simulink model "constantTorqueDemo"  (Simulink 8.3)
settings: Solver=ode45  StartTime=0.0  StopTime=inf  RelTol=1e-3
undefined symbols (not defined in the file or in its folder): PendulumPlant, PendulumVisualizer
libraries: drake x3, simulink x3
settings Model: Creator=russt  LastModifiedBy=russt
settings OptimizationCC: ExpressionDepthLimit=2147483647
settings DebuggingCC: FcnCallInpInsideContextMsg=UseLocalSettings

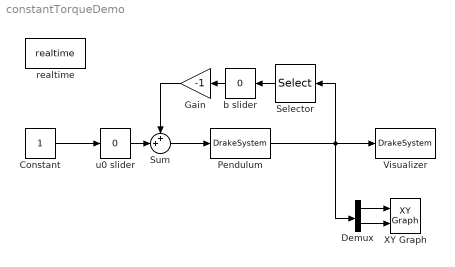
== system constantTorqueDemo ==
  Constant : Constant
  Demux : Demux  Outputs=2
  Gain : Gain  Gain=-1
  Pendulum : drake/DrakeSystem  sysobj=PendulumPlant(0)
  Selector : Selector  InputPortWidth=2  Indices=2
  Sum : Sum  Inputs=++|
  Visualizer : drake/DrakeSystem  sysobj=PendulumVisualizer()
  XY Graph : simulink/Sinks/XY Graph  xmin=-pi  xmax=pi  ymin=-4  ymax=4  st=-1
  "b slider " : simulink/Math Operations/Slider Gain  low=-5  gain=0  high=5
  realtime : drake/realtime  sample_time=.05  speed=1
  u0 slider : simulink/Math Operations/Slider Gain  low=-5  gain=0  high=5
  wires:
  Pendulum/1 -> Visualizer/1, Selector/1, Demux/1
  Constant/1 -> u0 slider/1
  Demux/1 -> XY Graph/1
  Demux/2 -> XY Graph/2
  Selector/1 -> "b slider "/1
  u0 slider/1 -> Sum/2
  Sum/1 -> Pendulum/1
  "b slider "/1 -> Gain/1
  Gain/1 -> Sum/1
